simulink model "ERES_PIMC_Controller_Simulation"  (R2018a)
settings: Solver=VariableStepAuto  StartTime=0.0  StopTime=120  RelTol=1e-3
undefined symbols (not defined in the file): a_lateral_max, atableall, feedback_filter_limit_max, feedback_filter_limit_min, fl_x, fl_y, fr_x, fr_y, friction_table, imc_acc_error_coeffi, integrator_saturation_level, Ki, num, proportion, proportion_loop_limit, speed_controller_input_limit, station_error_limit, station_integrator_saturation_level, station_Ki, station_Kp, steer_angle_limited, steer_ratio, T7_with_trailer_atable, T7_with_trailer_atableall, T7_with_trailer_engine_speed_table, T7_with_trailer_engine_throttle_table, T7_with_trailer_engine_torqe_tableall, T7_with_trailer_utable, T7_with_trailer_utableall, T7_with_trailer_vtable, t_delay, throttle_table, utable, v_table, Vr, vtable, w1, w2, wheel_base, x0, y0
libraries: simulink x2, Solver_SF x1
(part 1 of 2)
settings Model: SimulationMode=rapid-accelerator  Creator=DELL  LastModifiedBy=DELL

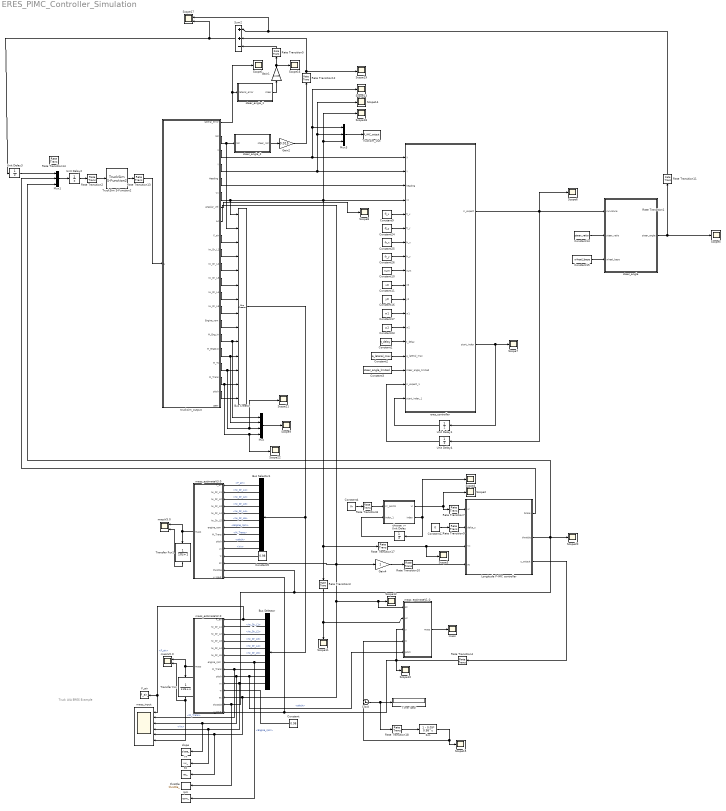
== system ERES_PIMC_Controller_Simulation ==
  note: Truck LKA ERES Example
  Bus Creator : BusCreator  Inputs=14
  Bus Selector : BusSelector  OutputSignals=F_air,Iw_Dr_L1,Iw_Dr_L2,Iw_Dr_L3,Iw_Dr_L4,Iw_Dr_L5,Engine_rpm,M_Trans,pitch,Vx
  Bus Selector1 : BusSelector  OutputSignals=F_air,Iw_Dr_L1,Iw_Dr_L2,Iw_Dr_L3,Iw_Dr_L4,Iw_Dr_L5,Engine_rpm,M_Trans,pitch,Vx
  Clock : Clock
  Constant : Constant  Value=0.98
  Constant1 : Constant  Value=t_delay
  Constant10 : Constant  Value=num
  Constant11 : Constant  Value=x0
  Constant12 : Constant  Value=0
  Constant14 : Constant  Value=steer_ratio
  Constant15 : Constant  Value=wheel_base
  Constant16 : Constant  Value=y0
  Constant17 : Constant  Value=w1
  Constant2 : Constant  Value=a_lateral_max
  Constant23 : Constant  Value=w2
  Constant24 : Constant  Value=fl_y
  Constant25 : Constant  Value=fr_x
  Constant26 : Constant  Value=fr_y
  Constant3 : Constant  Value=steer_angle_limited
  Constant4 : Constant  Value=Vr
  Constant5 : Constant  Value=0.98
  Constant9 : Constant  Value=fl_x
  F_air : ToWorkspace  VariableName=F_air_  SampleTime=0.01
  Fcn : Fcn  Expr=1 - 0.05* 0.98^u
  Gain1 : Gain  Gain=0.009
  Gain2 : Gain  Gain=0.015
  Gain4 : Gain
  Longitude P-IMC controller : Subsystem
  Mux : Mux
  Mux1 : Mux  Inputs=3
  Mux3 : Mux  Inputs=3
  Rate Transition{1,3..5,7..14,17..18} (14 alike) : RateTransition  OutPortSampleTime=0.01
  Rate Transition2 : RateTransition  OutPortSampleTime=0.001
  Scope{1..16,18..22} (21 alike) : Scope
  Scope17 : Scope  NumInputPorts=2
  Sum2 : Sum  Inputs=++-
  Time (sec) : Display
      settings: Format=bank  Decimation=100
  Transfer Fcn : TransferFcn  Denominator=[10 1]
  Transfer Fcn1 : TransferFcn  Denominator=[10 1]
  TruckSim S-Function2 : Solver_SF/TruckSim S-Function2  Priority=1  VehicleCode=s_ss__sss  SIMFILE=simfile.sim
      settings: AttributesFormatString=Vehicle Code: %<VehicleCode>
  Trucksim_Out : ToWorkspace  VariableName=P_IMC_output  SampleTime=-1
  Unit Delay : UnitDelay  InitialCondition=1  SampleTime=-1
  Unit Delay{1..4} (4 alike) : UnitDelay  SampleTime=0.01
  ac : ToWorkspace  VariableName=ac_  SampleTime=0.01
  choose_vr : MATLAB Function  TreatAsAtomicUnit=on
  eres_controller : MATLAB Function  TreatAsAtomicUnit=on
  mass : Scope
  massV2.0 : Scope  NumInputPorts=2
  massV3.0 : Scope  NumInputPorts=2
  mass_estimateV1.0 : Subsystem
  mass_estimateV2.0 : Subsystem
  mass_estimateV3.0 : Subsystem
  mass_input : Scope  NumInputPorts=6
  rpm : ToWorkspace  VariableName=rpm_  SampleTime=0.01
  slope : ToWorkspace  VariableName=slope_  SampleTime=0.01
  steer_angle : MATLAB Function  TreatAsAtomicUnit=on
  steer_angle_1 : Subsystem
  steer_angle_2 : Subsystem
  throttle : ToWorkspace  VariableName=throttle_  SampleTime=0.01
  trucksim_output : MATLAB Function  TreatAsAtomicUnit=on
  vx : ToWorkspace  VariableName=vx_  SampleTime=0.01
  wires:
  Constant1/1 -> eres_controller/14(t_delay)
  Constant3/1 -> eres_controller/16(steer_angle_limited)
  Unit Delay4/1 -> eres_controller/17(K_expect_1)
  TruckSim S-Function2/1 -> Rate Transition13/1
  Constant9/1 -> eres_controller/5(fl_x)
  Constant11/1 -> eres_controller/10(x0)
  eres_controller/2(start_index) -> Unit Delay1/1, Scope7/1
  Mux1/1 -> Unit Delay2/1
  Constant24/1 -> eres_controller/6(fl_y)
  Constant23/1 -> eres_controller/13(w2)
  Clock/1 -> Rate Transition18/1, Time (sec)/1
  Rate Transition8/1 -> choose_vr/1(Vr_points)
  Rate Transition7/1 -> Longitude P-IMC controller/1(vr)
  Unit Delay1/1 -> eres_controller/18(start_index_1)
  choose_vr/1(vr) -> Scope2/1, Rate Transition7/1
  Constant15/1 -> steer_angle/3(wheel_base)
  trucksim_output/8(Ac) -> mass_estimateV3.0/12(ac), mass_estimateV1.0/1(ac), Scope12/1, ac/1, mass_input/5, mass_estimateV2.0/12(ac), Gain4/1
  choose_vr/2(index) -> Unit Delay/1, Scope4/1
  Constant16/1 -> eres_controller/11(y0)
  Longitude P-IMC controller/2(throttle) -> throttle/1, mass_estimateV2.0/13(throttle), mass_estimateV3.0/13(throttle), Mux1/3, Scope20/1
  Constant25/1 -> eres_controller/7(fr_x)
  Constant4/1 -> Rate Transition8/1
  Rate Transition3/1 -> Scope11/1, mass_estimateV1.0/2(vc)
  Constant10/1 -> eres_controller/9(num)
  Longitude P-IMC controller/1(brake) -> Mux1/2
  Rate Transition18/1 -> Fcn/1
  Longitude P-IMC controller/3(u_output) -> Rate Transition4/1
  Rate Transition9/1 -> Longitude P-IMC controller/2(delta_s)
  Rate Transition13/1 -> trucksim_output/1(u)
  Constant17/1 -> eres_controller/12(w1)
  Unit Delay2/1 -> Rate Transition2/1
  Constant26/1 -> eres_controller/8(fr_y)
  Rate Transition2/1 -> TruckSim S-Function2/1
  eres_controller/1(K_expect) -> Scope6/1, steer_angle/1(curvature), Unit Delay4/1
  Constant14/1 -> steer_angle/2(steer_ratio)
  Rate Transition4/1 -> mass_estimateV3.0/14(u_input), mass_estimateV2.0/14(u_input), mass_estimateV1.0/3(u), Scope10/1
  trucksim_output/6(Vx) -> Bus Creator/1, Rate Transition17/1, Rate Transition3/1, Scope18/1, Mux3/3, eres_controller/4(vx)
  mass_estimateV1.0/1(mass) -> mass/1
  Rate Transition17/1 -> Longitude P-IMC controller/3(Vx), Scope3/1
  Constant12/1 -> Rate Transition9/1
  Unit Delay/1 -> choose_vr/2(index_1)
  Constant2/1 -> eres_controller/15(a_lateral_max)
  trucksim_output/7(angular_vel) -> Scope8/1
  Gain4/1 -> Rate Transition10/1
  steer_angle/1(steer_angle) -> Scope5/1, Rate Transition11/1
  Unit Delay3/1 -> Mux1/1
  Rate Transition10/1 -> Longitude P-IMC controller/4(ac)
  Mux3/1 -> Trucksim_Out/1
  trucksim_output/5(Heading) -> eres_controller/3(heading)
  trucksim_output/3(X) -> Mux3/1, Scope13/1, eres_controller/1(X)
  trucksim_output/4(Y) -> Mux3/2, Scope14/1, eres_controller/2(Y)
  trucksim_output/1(lateral_error) -> Scope1/1, steer_angle_1/1(lateral_error)
  Rate Transition5/1 -> Sum2/3
  Rate Transition11/1 -> Scope17/1, Sum2/1
  Sum2/1 -> Unit Delay3/1, Scope17/2
  steer_angle_1/1(steer) -> Gain1/1
  Gain1/1 -> Scope16/1, Rate Transition5/1
  trucksim_output/2(roll) -> Bus Creator/2, steer_angle_2/1(roll)
  steer_angle_2/1(steer_roll) -> Gain2/1
  Rate Transition12/1 -> Scope19/1, Sum2/2
  Gain2/1 -> Rate Transition12/1
  trucksim_output/19(M_Trans) -> Scope22/1, Mux/4, Bus Creator/13
  trucksim_output/18(M_Tc) -> Scope21/1, Mux/3, Bus Creator/12
  trucksim_output/17(M_EngOut) -> Mux/2, Bus Creator/11
  trucksim_output/16(M_Eng_In) -> Mux/1, Bus Creator/10
  trucksim_output/15(Engine_rpm) -> Bus Creator/9
  trucksim_output/14(Iw_Dr_L5) -> Bus Creator/8
  trucksim_output/13(Iw_Dr_L4) -> Bus Creator/7
  trucksim_output/12(Iw_Dr_L3) -> Bus Creator/6
  trucksim_output/11(Iw_Dr_L2) -> Bus Creator/5
  trucksim_output/10(Iw_Dr_L1) -> Bus Creator/4
  trucksim_output/9(F_air) -> Bus Creator/3
  Bus Creator/1 -> Bus Selector/1, Bus Selector1/1
  Bus Selector/1 -> F_air/1, mass_input/1, mass_estimateV2.0/1(F_air)  "<F_air>"
  Bus Selector/2 -> mass_estimateV2.0/2(Iw_Dr_L1)  "<Iw_Dr_L1>"
  Bus Selector/3 -> mass_estimateV2.0/3(Iw_Dr_L2)  "<Iw_Dr_L2>"
  Bus Selector/4 -> mass_estimateV2.0/4(Iw_Dr_L3)  "<Iw_Dr_L3>"
  Bus Selector/5 -> mass_estimateV2.0/5(Iw_Dr_L4)  "<Iw_Dr_L4>"
  Bus Selector/6 -> mass_estimateV2.0/6(Iw_Dr_L5)  "<Iw_Dr_L5>"
  Bus Selector/7 -> rpm/1, mass_estimateV2.0/7(engine_rpm)  "<Engine_rpm>"
  Bus Selector/8 -> mass_input/2, mass_estimateV2.0/8(M_Trans)  "<M_Trans>"
  Bus Selector/9 -> mass_estimateV1.0/5(pitch), slope/1, mass_input/3, mass_estimateV2.0/9(pitch)  "<pitch>"
  Bus Selector/10 -> vx/1, mass_input/4, mass_estimateV2.0/10(vx)  "<Vx>"
  Fcn/1 -> Scope15/1, mass_estimateV1.0/4(w)
  mass_estimateV2.0/1(mass) -> massV2.0/1, Transfer Fcn/1
  trucksim_output/20(pitch) -> Bus Creator/14
  Mux/1 -> Scope9/1
  Transfer Fcn/1 -> massV2.0/2, mass_input/6
  Constant/1 -> mass_estimateV2.0/11(w)
  Bus Selector1/1 -> mass_estimateV3.0/1(F_air)  "<F_air>"
  Bus Selector1/2 -> mass_estimateV3.0/2(Iw_Dr_L1)  "<Iw_Dr_L1>"
  Bus Selector1/3 -> mass_estimateV3.0/3(Iw_Dr_L2)  "<Iw_Dr_L2>"
  Bus Selector1/4 -> mass_estimateV3.0/4(Iw_Dr_L3)  "<Iw_Dr_L3>"
  Bus Selector1/5 -> mass_estimateV3.0/5(Iw_Dr_L4)  "<Iw_Dr_L4>"
  Bus Selector1/6 -> mass_estimateV3.0/6(Iw_Dr_L5)  "<Iw_Dr_L5>"
  Bus Selector1/7 -> mass_estimateV3.0/7(engine_rpm)  "<Engine_rpm>"
  Bus Selector1/8 -> mass_estimateV3.0/8(M_Trans)  "<M_Trans>"
  Bus Selector1/9 -> mass_estimateV3.0/9(pitch)  "<pitch>"
  Bus Selector1/10 -> mass_estimateV3.0/10(vx)  "<Vx>"
  Constant5/1 -> mass_estimateV3.0/11(w)
  Transfer Fcn1/1 -> massV3.0/2
  mass_estimateV3.0/1(mass) -> Transfer Fcn1/1, massV3.0/1

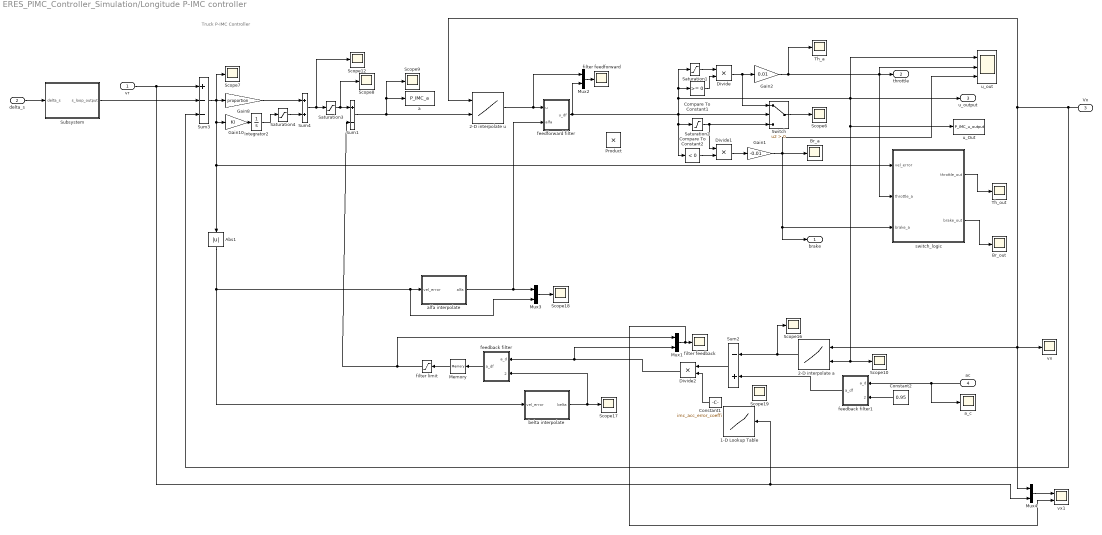
== system ERES_PIMC_Controller_Simulation/Longitude P-IMC controller ==
  note: Truck P-IMC Controller
  vr : Inport
  delta_s : Inport  Port=2
  Vx : Inport  Port=3
  ac : Inport  Port=4
  1-D Lookup Table : Lookup_n-D  NumberOfTableDimensions=1  BreakpointsForDimension1=[5 8 15 20 25 30]  Table=[0.3 0.45 0.65 0.8 0.9 1.0]  InternalRulePriority=Speed  RndMeth=Simplest  InputSameDT=on
  2-D interpolate a : Lookup_n-D  BreakpointsForDimension1=T7_with_trailer_vtable  BreakpointsForDimension2=T7_with_trailer_utable  Table=T7_with_trailer_atableall  ExtrapMethod=Clip  InternalRulePriority=Speed  RndMeth=Simplest  InputSameDT=on
  2-D interpolate u : Lookup_n-D  BreakpointsForDimension1=T7_with_trailer_vtable  BreakpointsForDimension2=T7_with_trailer_atable  Table=T7_with_trailer_utableall  ExtrapMethod=Clip  InternalRulePriority=Speed  RndMeth=Simplest  InputSameDT=on
  Abs1 : Abs
  Br_a : Scope
  Br_out : Scope
  Compare To Constant1 : simulink/Logic and Bit Operations/Compare To Constant  relop=>=  const=0  OutDataTypeStr=boolean
  Compare To Constant2 : simulink/Logic and Bit Operations/Compare To Constant  relop=<  const=0  OutDataTypeStr=boolean
  Constant1 : Constant  Value=imc_acc_error_coeffi
  Constant2 : Constant  Value=0.95
  Divide : Product  Inputs=**
  Divide1 : Product  Inputs=**
  Divide2 : Product  Inputs=**
  Gain1 : Gain  Gain=-0.01
  Gain10 : Gain  Gain=Ki
  Gain2 : Gain  Gain=0.01
  Gain8 : Gain  Gain=proportion
  Integrator2 : Integrator
  Memory : Memory
  Mux{1..4} (4 alike) : Mux  Inputs=2
  Product : Product
  Saturation1 : Saturate  UpperLimit=90  LowerLimit=0
  Saturation2 : Saturate  UpperLimit=0  LowerLimit=-60
  Saturation3 : Saturate  UpperLimit=proportion_loop_limit  LowerLimit=-proportion_loop_limit
  Saturation4 : Saturate  UpperLimit=integrator_saturation_level  LowerLimit=-integrator_saturation_level
  Scope{6..10,12,16..19} (10 alike) : Scope
  Subsystem : Subsystem
  Sum1 : Sum  Inputs=+-
  Sum2 : Sum  Inputs=-+
  Sum3 : Sum  Inputs=+--
  Sum4 : Sum
  Switch : Switch  Criteria=u2 > Threshold
  Th_a : Scope
  Th_out : Scope
  a : ToWorkspace  VariableName=P_IMC_a  SampleTime=0.01
  a_c : Scope
  alfa interpolate : MATLAB Function  TreatAsAtomicUnit=on
  belta interpolate : MATLAB Function  TreatAsAtomicUnit=on
  feedback filter : Subsystem
  feedback filter1 : Subsystem
  feedforward filter : Subsystem
  filter feedback : Scope
  filter feedforward : Scope
  filter limit : Saturate  UpperLimit=feedback_filter_limit_max  LowerLimit=feedback_filter_limit_min
  switch_logic : Subsystem
  u_Out : ToWorkspace  VariableName=P_IMC_u_output  SampleTime=0.01
  u_out : Scope  NumInputPorts=3
  vx : Scope
  vx1 : Scope  NumInputPorts=2
  brake : Outport
  throttle : Outport  Port=2
  u_output : Outport  Port=3
  wires:
  Vx/1 -> 2-D interpolate u/1, Mux4/1, 2-D interpolate a/1, vx/1, Sum3/3
  Sum1/1 -> a/1, Scope9/1, 2-D interpolate u/2
  Divide1/1 -> Gain1/1
  Compare To Constant2/1 -> Divide1/2
  Divide/1 -> Switch/1, Gain2/1
  Compare To Constant1/1 -> Divide/2
  Saturation1/1 -> Divide/1
  2-D interpolate u/1 -> Mux2/1, feedforward filter/1(u)
  Gain1/1 -> u_out/3, switch_logic/3(brake_a), brake/1, Br_a/1
  Gain2/1 -> u_out/2, throttle/1, switch_logic/2(throttle_a), Th_a/1
  Switch/1 -> Scope6/1
  Saturation2/1 -> Switch/3, Divide1/1
  Sum3/1 -> Gain8/1, Scope7/1, Gain10/1, switch_logic/1(vel_error), Abs1/1
  Saturation3/1 -> Scope8/1, Sum1/1
  delta_s/1 -> Subsystem/1(delta_s)
  Subsystem/1(s_loop_output) -> Sum3/2
  ac/1 -> a_c/1, feedback filter1/1(a_d)
  Sum4/1 -> Scope12/1, Saturation3/1
  Gain8/1 -> Sum4/1
  Gain10/1 -> Integrator2/1
  Mux1/1 -> vx1/2, filter feedback/1
  feedback filter/1(a_df) -> Memory/1
  Memory/1 -> filter limit/1
  2-D interpolate a/1 -> Sum2/1, Scope16/1
  filter limit/1 -> Sum1/2, Mux1/1
  alfa interpolate/1(alfa) -> Mux3/1, feedforward filter/2(alfa)
  Abs1/1 -> Mux3/2, alfa interpolate/1(vel_error), belta interpolate/1(vel_error)
  Mux3/1 -> Scope18/1
  Mux2/1 -> filter feedforward/1
  belta interpolate/1(belta) -> feedback filter/2(belta), Scope17/1
  vr/1 -> 1-D Lookup Table/1, Mux4/2, Sum3/1
  Sum2/1 -> Divide2/1
  Divide2/1 -> Mux1/2, feedback filter/1(a_d)
  feedforward filter/1(u_df) -> Compare To Constant1/1, Saturation1/1, u_out/1, u_Out/1, Scope10/1, 2-D interpolate a/2, u_output/1, Saturation2/1, Compare To Constant2/1, Switch/2, Mux2/2
  switch_logic/1(throttle_out) -> Th_out/1
  switch_logic/2(brake_out) -> Br_out/1
  Constant2/1 -> feedback filter1/2(belta)
  feedback filter1/1(a_df) -> Sum2/2
  Mux4/1 -> vx1/1
  Integrator2/1 -> Saturation4/1
  Saturation4/1 -> Sum4/2
  Constant1/1 -> Divide2/2

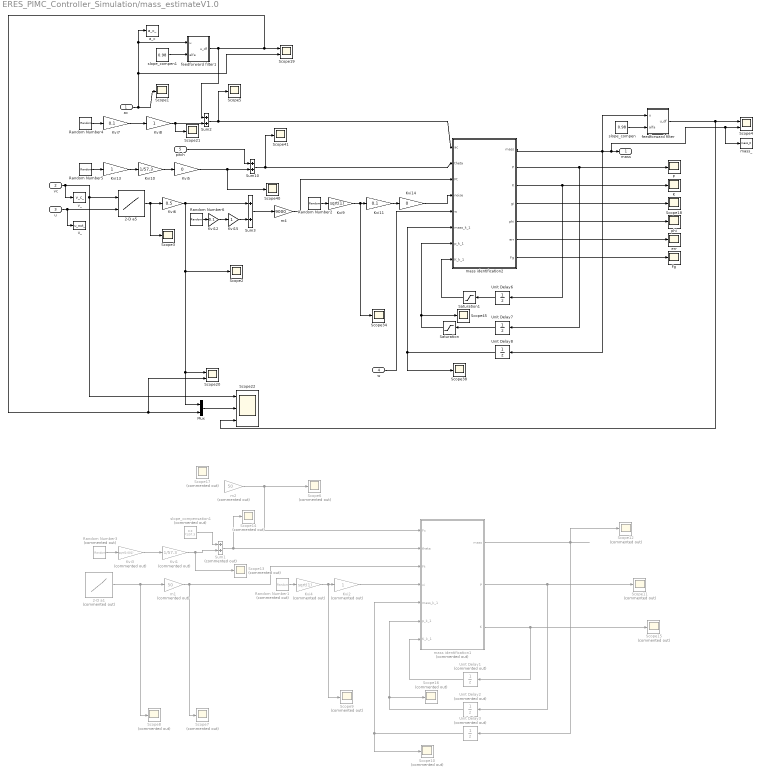
== system ERES_PIMC_Controller_Simulation/mass_estimateV1.0 ==
  ac : Inport
  vc : Inport  Port=2
  u : Inport  Port=3
  w : Inport  Port=4
  pitch : Inport  Port=5
  2-D a1 : Lookup_n-D  Commented=on  BreakpointsForDimension1=vtable  BreakpointsForDimension2=utable  BreakpointsForDimension3=[-60 -50]  Table=atableall  InternalRulePriority=Speed  RndMeth=Simplest  InputSameDT=on
  2-D a5 : Lookup_n-D  BreakpointsForDimension1=T7_with_trailer_vtable  BreakpointsForDimension2=T7_with_trailer_utable  BreakpointsForDimension3=[-60 -50]  Table=T7_with_trailer_atableall  InternalRulePriority=Speed  RndMeth=Simplest  InputSameDT=on
  Fg : Scope
  K : Scope
  Kvi1 : Gain  Commented=on  Gain=1/57.3
  Kvi10 : Gain  Gain=1/57.3
  Kvi11 : Gain  Gain=0.1
  Kvi12 : Gain  Gain=0.1
  Kvi13 : Gain
  Kvi14 : Gain  Gain=0
  Kvi15 : Gain
  Kvi2 : Gain  Commented=on
  Kvi3 : Gain  Commented=on  Gain=sqrt(0.001)
  Kvi4 : Gain  Commented=on  Gain=sqrt(1)
  Kvi5 : Gain  Gain=0
  Kvi6 : Gain  Gain=0.5
  Kvi7 : Gain  Gain=0.1
  Kvi8 : Gain
  Kvi9 : Gain  Gain=sqrt(1)
  Mux : Mux  Inputs=2
  P : Scope
  Random Number1 : RandomNumber  Commented=on  SampleTime=0.01
  Random Number{2,4..6} (4 alike) : RandomNumber  SampleTime=0.01
  Random Number3 : RandomNumber  Commented=on  Variance=0.1  SampleTime=0.01
  Saturation : Saturate  UpperLimit=10000000  LowerLimit=0.02
  Saturation1 : Saturate  UpperLimit=100  LowerLimit=0.1
  Scope{1..3,5,18,21,34,38,40..41,45} (11 alike) : Scope
  Scope{6..17} (12 alike) : Scope  Commented=on
  Scope19 : Scope  NumInputPorts=2
  Scope20 : Scope  NumInputPorts=2
  Scope22 : Scope  NumInputPorts=3
  Scope4 : Scope  NumInputPorts=2
  Sum1 : Sum  Commented=on
  Sum10 : Sum
  Sum2 : Sum
  Sum3 : Sum
  Unit Delay1 : UnitDelay  Commented=on  InitialCondition=1  SampleTime=0.01
  Unit Delay2 : UnitDelay  Commented=on  InitialCondition=100000  SampleTime=0.01
  Unit Delay3 : UnitDelay  Commented=on  InitialCondition=30000  SampleTime=0.01
  Unit Delay6 : UnitDelay  InitialCondition=10  SampleTime=0.01
  Unit Delay7 : UnitDelay  InitialCondition=100000  SampleTime=0.01
  Unit Delay8 : UnitDelay  InitialCondition=40000  SampleTime=0.01
  a_c : ToWorkspace  VariableName=a_c_  SampleTime=0.01
  err : Scope
  feedforward filter : Subsystem
  feedforward filter1 : Subsystem
  m1 : Gain  Commented=on  Gain=50
  m2 : Gain  Commented=on  Gain=50
  m4 : Gain  Gain=9000
  mass identification1 : MATLAB Function  Commented=on  TreatAsAtomicUnit=on  SystemSampleTime=0.01
  mass identification2 : MATLAB Function  TreatAsAtomicUnit=on  SystemSampleTime=0.01
  mass_ : ToWorkspace  VariableName=mass_0  SampleTime=0.01
  phi : Scope
  slope_compen : Constant  Value=0.98
  slope_compen1 : Constant  Value=0.98
  slope_compensation1 : Constant  Commented=on  Value=0.0 *1/57.3
  u_ : ToWorkspace  VariableName=u_out_  SampleTime=0.01
  v_ : ToWorkspace  VariableName=v_c_  SampleTime=0.01
  mass : Outport
  wires:
  Unit Delay7/1 -> Saturation/1
  mass identification2/1(mass) -> feedforward filter/1(u), Unit Delay8/1, mass_/1, Scope4/2, mass/1
  mass identification2/3(K) -> Unit Delay6/1, K/1
  Unit Delay6/1 -> Saturation1/1
  Kvi13/1 -> Kvi10/1
  Kvi11/1 -> Kvi14/1
  Random Number2/1 -> Kvi9/1
  Unit Delay8/1 -> mass identification2/6(mass_k_1), Scope38/1
  pitch/1 -> Sum10/1
  Kvi10/1 -> Kvi5/1
  Random Number5/1 -> Kvi13/1
  mass identification2/2(P) -> Unit Delay7/1, P/1
  vc/1 -> v_/1, Scope22/1, 2-D a5/1
  Kvi9/1 -> Kvi11/1, Scope34/1
  Sum10/1 -> mass identification2/2(theta), Scope41/1
  u/1 -> u_/1, 2-D a5/2
  m2/1 -> Scope6/1, mass identification1/1(Fc)
  ? -> 2-D a1/2
  m1/1 -> mass identification1/3(Ft), Scope7/1
  Sum1/1 -> Scope14/1, mass identification1/2(theta)
  Kvi4/1 -> Scope9/1, Kvi2/1
  ? -> 2-D a1/1
  2-D a1/1 -> m1/1, Scope8/1
  mass identification1/2(P) -> Scope11/1, Unit Delay2/1
  Random Number3/1 -> Kvi3/1
  Kvi1/1 -> Scope13/1, Sum1/2
  slope_compensation1/1 -> Sum1/1
  Unit Delay3/1 -> Scope10/1, mass identification1/5(mass_k_1)
  Random Number1/1 -> Kvi4/1
  Kvi2/1 -> mass identification1/4(xi)
  ? -> m2/1, Scope17/1
  Kvi3/1 -> Kvi1/1
  Unit Delay1/1 -> mass identification1/7(K_k_1)
  mass identification1/3(K) -> Scope15/1, Unit Delay1/1
  mass identification1/1(mass) -> Unit Delay3/1, Scope12/1
  Unit Delay2/1 -> Scope16/1, mass identification1/6(p_k_1)
  mass identification2/4(gi) -> Scope18/1
  mass identification2/5(phi) -> phi/1
  Kvi5/1 -> Scope40/1, Sum10/2
  Random Number4/1 -> Kvi7/1
  Kvi7/1 -> Kvi8/1
  Kvi8/1 -> Scope21/1, Sum2/2
  w/1 -> mass identification2/5(w)
  feedforward filter/1(u_df) -> Scope22/3, Scope4/1
  slope_compen/1 -> feedforward filter/2(alfa)
  2-D a5/1 -> Scope3/1, Kvi6/1
  Sum2/1 -> mass identification2/1(ac), Scope5/1
  mass identification2/6(err) -> err/1
  Saturation/1 -> mass identification2/7(p_k_1), Scope45/1
  Saturation1/1 -> mass identification2/8(K_k_1)
  slope_compen1/1 -> feedforward filter1/2(alfa)
  feedforward filter1/1(u_df) -> Sum2/1, Scope20/2, Mux/2, Scope19/1
  ac/1 -> Scope1/1, Scope19/2, feedforward filter1/1(u), a_c/1
  Mux/1 -> Scope22/2
  Random Number6/1 -> Kvi12/1
  Kvi12/1 -> Kvi15/1
  Sum3/1 -> m4/1
  Kvi6/1 -> Scope2/1, Scope20/1, Mux/1, Sum3/1
  m4/1 -> mass identification2/3(Ft)
  mass identification2/7(Fg) -> Fg/1
  Kvi14/1 -> mass identification2/4(noise)
  Kvi15/1 -> Sum3/2

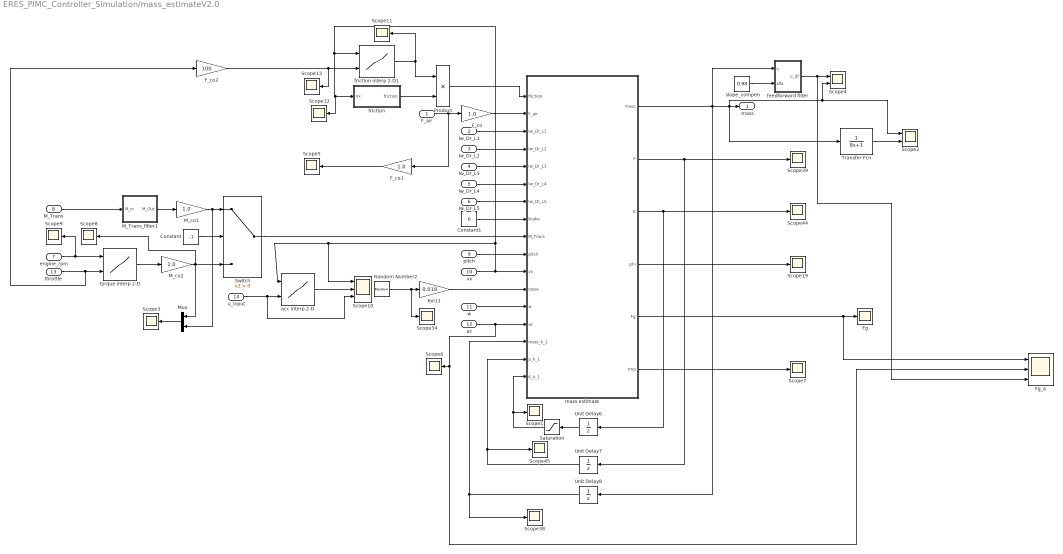
== system ERES_PIMC_Controller_Simulation/mass_estimateV2.0 ==
  F_air : Inport
  Iw_Dr_L1 : Inport  Port=2
  Iw_Dr_L2 : Inport  Port=3
  Iw_Dr_L3 : Inport  Port=4
  Iw_Dr_L4 : Inport  Port=5
  Iw_Dr_L5 : Inport  Port=6
  engine_rpm : Inport  Port=7
  M_Trans : Inport  Port=8
  pitch : Inport  Port=9
  vx : Inport  Port=10
  w : Inport  Port=11
  ac : Inport  Port=12
  throttle : Inport  Port=13
  u_input : Inport  Port=14
  Constant : Constant  Value=-1
  Constant1 : Constant  Value=0
  F_co : Gain  Gain=1.0
  F_co1 : Gain  Gain=1.0
  F_co2 : Gain  Gain=100
  Fg : Scope
  Fg_a : Scope  NumInputPorts=3
  Kvi11 : Gain  Gain=0.018
  M_Trans_filter1 : Subsystem
  M_co1 : Gain  Gain=1.0
  M_co2 : Gain  Gain=1.0
  Mux : Mux  Inputs=2
  Product : Product
  Random Number2 : RandomNumber  SampleTime=0.01
  Saturation : Saturate  UpperLimit=10  LowerLimit=0.01
  Scope{1,3,5..9,11..13,19,34,38..39,44..45} (16 alike) : Scope
  Scope10 : Scope  NumInputPorts=3
  Scope2 : Scope  NumInputPorts=2
  Scope4 : Scope  NumInputPorts=2
  Switch : Switch  Criteria=u2 > Threshold
  Transfer Fcn : TransferFcn  Denominator=[8 1]
  Unit Delay6 : UnitDelay  SampleTime=0.01
  Unit Delay7 : UnitDelay  InitialCondition=1000000  SampleTime=0.01
  Unit Delay8 : UnitDelay  InitialCondition=40000  SampleTime=0.01
  acc interp 2-D : Lookup_n-D  BreakpointsForDimension1=T7_with_trailer_vtable  BreakpointsForDimension2=T7_with_trailer_utable  BreakpointsForDimension3=[-60 -50]  Table=T7_with_trailer_atableall  InternalRulePriority=Speed  RndMeth=Simplest  InputSameDT=on
  feedforward filter : Subsystem
  friction : Subsystem
  friction interp 2-D1 : Lookup_n-D  BreakpointsForDimension1=v_table  BreakpointsForDimension2=throttle_table  BreakpointsForDimension3=[-60 -50]  Table=friction_table  InternalRulePriority=Speed  RndMeth=Simplest  InputSameDT=on
  mass estimate : MATLAB Function  TreatAsAtomicUnit=on  SystemSampleTime=0.01
  slope_compen : Constant  Value=0.98
  "torque interp 2-D " : Lookup_n-D  BreakpointsForDimension1=T7_with_trailer_engine_speed_table  BreakpointsForDimension2=T7_with_trailer_engine_throttle_table  BreakpointsForDimension3=[-60 -50]  Table=T7_with_trailer_engine_torqe_tableall  InternalRulePriority=Speed  RndMeth=Simplest  InputSameDT=on
  mass : Outport
  wires:
  slope_compen/1 -> feedforward filter/2(alfa)
  feedforward filter/1(u_df) -> Fg_a/3, Scope4/1
  mass estimate/4(phi) -> Scope19/1
  Random Number2/1 -> Scope34/1, Kvi11/1
  mass estimate/2(P) -> Unit Delay7/1, Scope39/1
  Unit Delay6/1 -> Saturation/1
  mass estimate/3(K) -> Unit Delay6/1, Scope44/1
  mass estimate/1(mass) -> Unit Delay8/1, Transfer Fcn/1, mass/1, Scope2/1, Scope4/2, feedforward filter/1(u)
  Unit Delay7/1 -> Scope45/1, mass estimate/16(p_k_1)
  Iw_Dr_L5/1 -> mass estimate/7(Iw_Dr_L5)
  Iw_Dr_L4/1 -> mass estimate/6(Iw_Dr_L4)
  Iw_Dr_L3/1 -> mass estimate/5(Iw_Dr_L3)
  Iw_Dr_L2/1 -> mass estimate/4(Iw_Dr_L2)
  Iw_Dr_L1/1 -> mass estimate/3(Iw_Dr_L1)
  F_air/1 -> F_co1/1, F_co/1
  w/1 -> mass estimate/13(w)
  vx/1 -> Scope10/1, acc interp 2-D/1, friction interp 2-D1/1, Scope12/1, friction/1(Vx), mass estimate/11(vx)
  ac/1 -> Fg_a/2, Scope6/1, mass estimate/14(ac)
  Unit Delay8/1 -> Scope38/1, mass estimate/15(mass_k_1)
  Saturation/1 -> Scope1/1, mass estimate/17(K_k_1)
  mass estimate/6(tmp) -> Scope7/1
  mass estimate/5(Fg) -> Fg_a/1, Fg/1
  pitch/1 -> mass estimate/10(pitch)
  Switch/1 -> mass estimate/9(M_Trans)
  F_co/1 -> mass estimate/2(F_air)
  friction/1(friction) -> Product/2
  Product/1 -> mass estimate/1(friction)
  Transfer Fcn/1 -> Scope2/2
  F_co1/1 -> Scope5/1
  Constant/1 -> Switch/2
  M_Trans_filter1/1(M_Out) -> M_co1/1
  M_co1/1 -> Mux/2, Switch/1
  "torque interp 2-D "/1 -> M_co2/1
  engine_rpm/1 -> Scope9/1, "torque interp 2-D "/1
  throttle/1 -> F_co2/1, "torque interp 2-D "/2
  M_Trans/1 -> M_Trans_filter1/1(M_in)
  M_co2/1 -> Scope8/1, Mux/1, Switch/3
  Mux/1 -> Scope3/1
  Constant1/1 -> mass estimate/8(brake)
  acc interp 2-D/1 -> Scope10/2
  u_input/1 -> Scope10/3, acc interp 2-D/2
  F_co2/1 -> friction interp 2-D1/2, Scope13/1
  friction interp 2-D1/1 -> Product/1, Scope11/1
  Kvi11/1 -> mass estimate/12(noise)

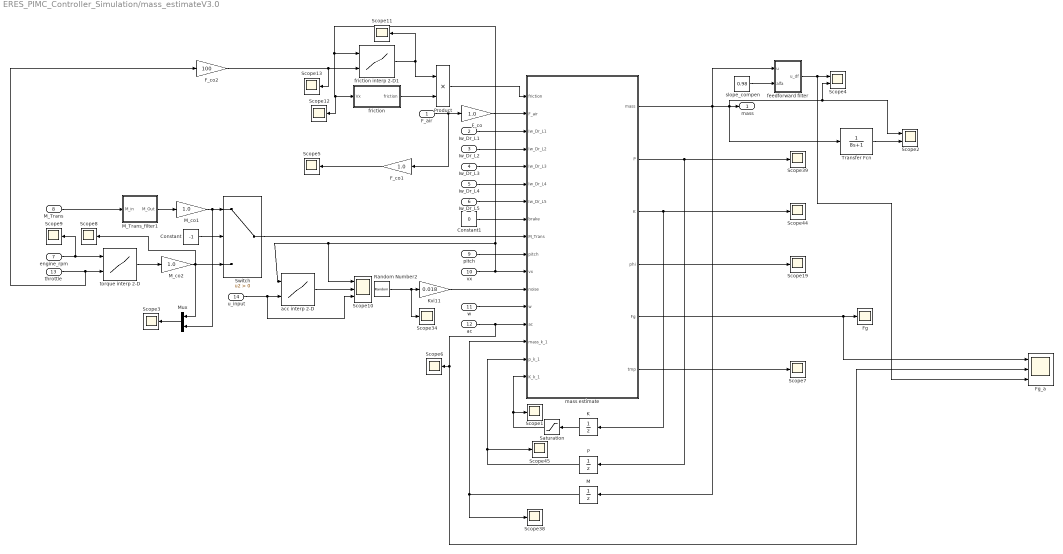
== system ERES_PIMC_Controller_Simulation/mass_estimateV3.0 ==
  F_air : Inport
  Iw_Dr_L1 : Inport  Port=2
  Iw_Dr_L2 : Inport  Port=3
  Iw_Dr_L3 : Inport  Port=4
  Iw_Dr_L4 : Inport  Port=5
  Iw_Dr_L5 : Inport  Port=6
  engine_rpm : Inport  Port=7
  M_Trans : Inport  Port=8
  pitch : Inport  Port=9
  vx : Inport  Port=10
  w : Inport  Port=11
  ac : Inport  Port=12
  throttle : Inport  Port=13
  u_input : Inport  Port=14
  Constant : Constant  Value=-1
  Constant1 : Constant  Value=0
  F_co : Gain  Gain=1.0
  F_co1 : Gain  Gain=1.0
  F_co2 : Gain  Gain=100
  Fg : Scope
  Fg_a : Scope  NumInputPorts=3
  K : UnitDelay  SampleTime=0.01
  Kvi11 : Gain  Gain=0.018
  M : UnitDelay  InitialCondition=40000  SampleTime=0.01
  M_Trans_filter1 : Subsystem
  M_co1 : Gain  Gain=1.0
  M_co2 : Gain  Gain=1.0
  Mux : Mux  Inputs=2
  P : UnitDelay  InitialCondition=1000000  SampleTime=0.01
  Product : Product
  Random Number2 : RandomNumber  SampleTime=0.01
  Saturation : Saturate  UpperLimit=10  LowerLimit=0.01
  Scope{1,3,5..9,11..13,19,34,38..39,44..45} (16 alike) : Scope
  Scope10 : Scope  NumInputPorts=3
  Scope2 : Scope  NumInputPorts=2
  Scope4 : Scope  NumInputPorts=2
  Switch : Switch  Criteria=u2 > Threshold
  Transfer Fcn : TransferFcn  Denominator=[8 1]
  acc interp 2-D : Lookup_n-D  BreakpointsForDimension1=T7_with_trailer_vtable  BreakpointsForDimension2=T7_with_trailer_utable  BreakpointsForDimension3=[-60 -50]  Table=T7_with_trailer_atableall  InternalRulePriority=Speed  RndMeth=Simplest  InputSameDT=on
  feedforward filter : Subsystem
  friction : Subsystem
  friction interp 2-D1 : Lookup_n-D  BreakpointsForDimension1=v_table  BreakpointsForDimension2=throttle_table  BreakpointsForDimension3=[-60 -50]  Table=friction_table  InternalRulePriority=Speed  RndMeth=Simplest  InputSameDT=on
  mass estimate : MATLAB Function  TreatAsAtomicUnit=on  SystemSampleTime=0.01
  slope_compen : Constant  Value=0.98
  "torque interp 2-D " : Lookup_n-D  BreakpointsForDimension1=T7_with_trailer_engine_speed_table  BreakpointsForDimension2=T7_with_trailer_engine_throttle_table  BreakpointsForDimension3=[-60 -50]  Table=T7_with_trailer_engine_torqe_tableall  InternalRulePriority=Speed  RndMeth=Simplest  InputSameDT=on
  mass : Outport
  wires:
  Kvi11/1 -> mass estimate/12(noise)
  friction interp 2-D1/1 -> Scope11/1, Product/1
  F_co2/1 -> Scope13/1, friction interp 2-D1/2
  u_input/1 -> acc interp 2-D/2, Scope10/3
  acc interp 2-D/1 -> Scope10/2
  Constant1/1 -> mass estimate/8(brake)
  Mux/1 -> Scope3/1
  M_co2/1 -> Switch/3, Mux/1, Scope8/1
  M_Trans/1 -> M_Trans_filter1/1(M_in)
  throttle/1 -> "torque interp 2-D "/2, F_co2/1
  engine_rpm/1 -> "torque interp 2-D "/1, Scope9/1
  "torque interp 2-D "/1 -> M_co2/1
  M_co1/1 -> Switch/1, Mux/2
  M_Trans_filter1/1(M_Out) -> M_co1/1
  Constant/1 -> Switch/2
  F_co1/1 -> Scope5/1
  Transfer Fcn/1 -> Scope2/2
  Product/1 -> mass estimate/1(friction)
  friction/1(friction) -> Product/2
  F_co/1 -> mass estimate/2(F_air)
  Switch/1 -> mass estimate/9(M_Trans)
  pitch/1 -> mass estimate/10(pitch)
  mass estimate/5(Fg) -> Fg/1, Fg_a/1
  mass estimate/6(tmp) -> Scope7/1
  Saturation/1 -> mass estimate/17(K_k_1), Scope1/1
  M/1 -> mass estimate/15(mass_k_1), Scope38/1
  ac/1 -> mass estimate/14(ac), Scope6/1, Fg_a/2
  vx/1 -> mass estimate/11(vx), friction/1(Vx), Scope12/1, friction interp 2-D1/1, acc interp 2-D/1, Scope10/1
  w/1 -> mass estimate/13(w)
  F_air/1 -> F_co/1, F_co1/1
  Iw_Dr_L1/1 -> mass estimate/3(Iw_Dr_L1)
  Iw_Dr_L2/1 -> mass estimate/4(Iw_Dr_L2)
  Iw_Dr_L3/1 -> mass estimate/5(Iw_Dr_L3)
  Iw_Dr_L4/1 -> mass estimate/6(Iw_Dr_L4)
  Iw_Dr_L5/1 -> mass estimate/7(Iw_Dr_L5)
  P/1 -> mass estimate/16(p_k_1), Scope45/1
  mass estimate/1(mass) -> feedforward filter/1(u), Scope4/2, Scope2/1, mass/1, Transfer Fcn/1, M/1
  mass estimate/3(K) -> Scope44/1, K/1
  K/1 -> Saturation/1
  mass estimate/2(P) -> Scope39/1, P/1
  Random Number2/1 -> Kvi11/1, Scope34/1
  mass estimate/4(phi) -> Scope19/1
  feedforward filter/1(u_df) -> Scope4/1, Fg_a/3
  slope_compen/1 -> feedforward filter/2(alfa)

== system ERES_PIMC_Controller_Simulation/steer_angle_1 ==
  lateral_error : Inport
  steer_compensation : MATLAB Function  TreatAsAtomicUnit=on
  steer : Outport
  wires:
  lateral_error/1 -> steer_compensation/1(lateral_error)
  steer_compensation/1(steer_compensation) -> steer/1

== system ERES_PIMC_Controller_Simulation/steer_angle_2 ==
  roll : Inport
  steer_roll_compensation : MATLAB Function  TreatAsAtomicUnit=on
  steer_roll : Outport
  wires:
  steer_roll_compensation/1(steer_roll_) -> steer_roll/1
  roll/1 -> steer_roll_compensation/1(roll)

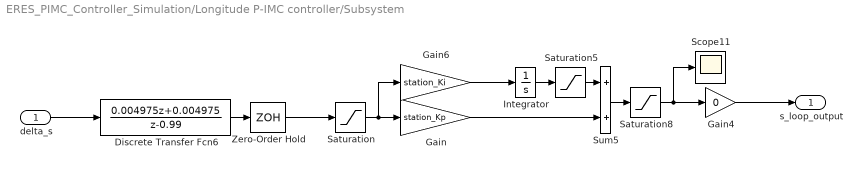
== system ERES_PIMC_Controller_Simulation/Longitude P-IMC controller/Subsystem ==
  delta_s : Inport
  Discrete Transfer Fcn6 : DiscreteTransferFcn  Numerator=[0.004975 0.004975]  Denominator=[1 -0.99]
  Gain : Gain  Gain=station_Kp
  Gain4 : Gain  Gain=0
  Gain6 : Gain  Gain=station_Ki
  Integrator : Integrator
  Saturation : Saturate  UpperLimit=station_error_limit  LowerLimit=-station_error_limit
  Saturation5 : Saturate  UpperLimit=station_integrator_saturation_level  LowerLimit=-station_integrator_saturation_level
  Saturation8 : Saturate  UpperLimit=speed_controller_input_limit  LowerLimit=-speed_controller_input_limit
  Scope11 : Scope
  Sum5 : Sum
  Zero-Order Hold : ZeroOrderHold  SampleTime=0.01
  s_loop_output : Outport
  wires:
  Sum5/1 -> Saturation8/1
  Gain6/1 -> Integrator/1
  Gain/1 -> Sum5/2
  Discrete Transfer Fcn6/1 -> Zero-Order Hold/1
  Saturation5/1 -> Sum5/1
  Saturation8/1 -> Gain4/1, Scope11/1
  Saturation/1 -> Gain/1, Gain6/1
  delta_s/1 -> Discrete Transfer Fcn6/1
  Integrator/1 -> Saturation5/1
  Zero-Order Hold/1 -> Saturation/1
  Gain4/1 -> s_loop_output/1

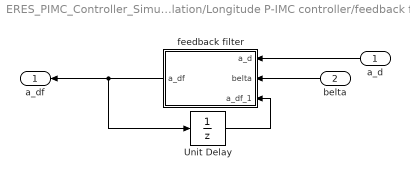
== system ERES_PIMC_Controller_Simulation/Longitude P-IMC controller/feedback filter ==
  a_d : Inport
  belta : Inport  Port=2
  Unit Delay : UnitDelay  SampleTime=-1
  feedback filter : MATLAB Function  TreatAsAtomicUnit=on
  a_df : Outport
  wires:
  Unit Delay/1 -> feedback filter/3(a_df_1)
  a_d/1 -> feedback filter/1(a_d)
  feedback filter/1(a_df) -> a_df/1, Unit Delay/1
  belta/1 -> feedback filter/2(belta)

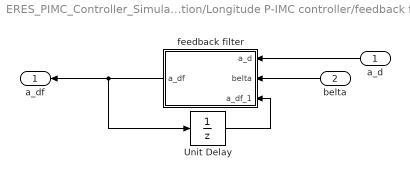
== system ERES_PIMC_Controller_Simulation/Longitude P-IMC controller/feedback filter1 ==
  a_d : Inport
  belta : Inport  Port=2
  Unit Delay : UnitDelay  SampleTime=-1
  feedback filter : MATLAB Function  TreatAsAtomicUnit=on
  a_df : Outport
  wires:
  belta/1 -> feedback filter/2(belta)
  feedback filter/1(a_df) -> Unit Delay/1, a_df/1
  a_d/1 -> feedback filter/1(a_d)
  Unit Delay/1 -> feedback filter/3(a_df_1)

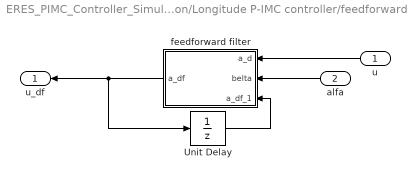
== system ERES_PIMC_Controller_Simulation/Longitude P-IMC controller/feedforward filter ==
  u : Inport
  alfa : Inport  Port=2
  Unit Delay : UnitDelay  SampleTime=-1
  feedforward filter : MATLAB Function  TreatAsAtomicUnit=on
  u_df : Outport
  wires:
  alfa/1 -> feedforward filter/2(belta)
  feedforward filter/1(a_df) -> Unit Delay/1, u_df/1
  u/1 -> feedforward filter/1(a_d)
  Unit Delay/1 -> feedforward filter/3(a_df_1)

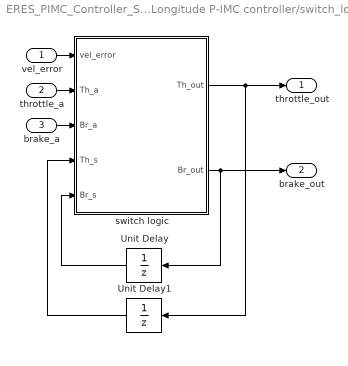
== system ERES_PIMC_Controller_Simulation/Longitude P-IMC controller/switch_logic ==
  vel_error : Inport
  throttle_a : Inport  Port=2
  brake_a : Inport  Port=3
  Unit Delay : UnitDelay  SampleTime=-1
  Unit Delay1 : UnitDelay  SampleTime=-1
  switch logic : MATLAB Function  TreatAsAtomicUnit=on
  throttle_out : Outport
  brake_out : Outport  Port=2
  wires:
  brake_a/1 -> switch logic/3(Br_a)
  switch logic/2(Br_out) -> brake_out/1, Unit Delay/1
  switch logic/1(Th_out) -> throttle_out/1, Unit Delay1/1
  Unit Delay1/1 -> switch logic/4(Th_s)
  Unit Delay/1 -> switch logic/5(Br_s)
  throttle_a/1 -> switch logic/2(Th_a)
  vel_error/1 -> switch logic/1(vel_error)

== system ERES_PIMC_Controller_Simulation/mass_estimateV1.0/feedforward filter ==
  u : Inport
  alfa : Inport  Port=2
  Unit Delay : UnitDelay  SampleTime=-1
  feedforward filter : MATLAB Function  TreatAsAtomicUnit=on
  u_df : Outport
  wires:
  alfa/1 -> feedforward filter/2(belta)
  feedforward filter/1(a_df) -> Unit Delay/1, u_df/1
  u/1 -> feedforward filter/1(a_d)
  Unit Delay/1 -> feedforward filter/3(a_df_1)

== system ERES_PIMC_Controller_Simulation/mass_estimateV1.0/feedforward filter1 ==
  u : Inport
  alfa : Inport  Port=2
  Unit Delay : UnitDelay  SampleTime=-1
  feedforward filter : MATLAB Function  TreatAsAtomicUnit=on
  u_df : Outport
  wires:
  Unit Delay/1 -> feedforward filter/3(a_df_1)
  u/1 -> feedforward filter/1(a_d)
  feedforward filter/1(a_df) -> u_df/1, Unit Delay/1
  alfa/1 -> feedforward filter/2(belta)

== system ERES_PIMC_Controller_Simulation/mass_estimateV2.0/M_Trans_filter1 ==
  M_in : Inport
  Scope3 : Scope  NumInputPorts=2
  feedforward filter1 : Subsystem
  slope_compen1 : Constant  Value=0.98
  M_Out : Outport
  wires:
  feedforward filter1/1(u_df) -> Scope3/1, M_Out/1
  slope_compen1/1 -> feedforward filter1/2(alfa)
  M_in/1 -> Scope3/2, feedforward filter1/1(u)

== system ERES_PIMC_Controller_Simulation/mass_estimateV2.0/feedforward filter ==
  u : Inport
  alfa : Inport  Port=2
  Unit Delay : UnitDelay  SampleTime=-1
  feedforward filter : MATLAB Function  TreatAsAtomicUnit=on
  u_df : Outport
  wires:
  Unit Delay/1 -> feedforward filter/3(a_df_1)
  u/1 -> feedforward filter/1(a_d)
  feedforward filter/1(a_df) -> u_df/1, Unit Delay/1
  alfa/1 -> feedforward filter/2(belta)

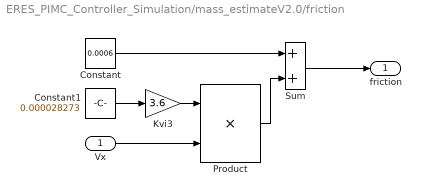
== system ERES_PIMC_Controller_Simulation/mass_estimateV2.0/friction ==
  Vx : Inport
  Constant : Constant  Value=0.0006
  Constant1 : Constant  Value=0.000028273
  Kvi3 : Gain  Gain=3.6
  Product : Product
  Sum : Sum
  friction : Outport
  wires:
  Vx/1 -> Product/2
  Sum/1 -> friction/1
  Constant1/1 -> Kvi3/1
  Product/1 -> Sum/2
  Constant/1 -> Sum/1
  Kvi3/1 -> Product/1

== system ERES_PIMC_Controller_Simulation/mass_estimateV3.0/M_Trans_filter1 ==
  M_in : Inport
  Scope3 : Scope  NumInputPorts=2
  feedforward filter1 : Subsystem
  slope_compen1 : Constant  Value=0.98
  M_Out : Outport
  wires:
  M_in/1 -> feedforward filter1/1(u), Scope3/2
  slope_compen1/1 -> feedforward filter1/2(alfa)
  feedforward filter1/1(u_df) -> M_Out/1, Scope3/1

== system ERES_PIMC_Controller_Simulation/mass_estimateV3.0/feedforward filter ==
  u : Inport
  alfa : Inport  Port=2
  Unit Delay : UnitDelay  SampleTime=-1
  feedforward filter : MATLAB Function  TreatAsAtomicUnit=on
  u_df : Outport
  wires:
  alfa/1 -> feedforward filter/2(belta)
  feedforward filter/1(a_df) -> Unit Delay/1, u_df/1
  u/1 -> feedforward filter/1(a_d)
  Unit Delay/1 -> feedforward filter/3(a_df_1)

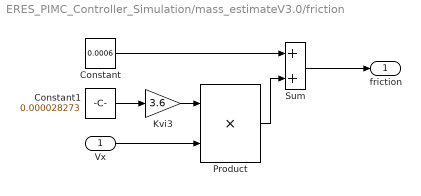
== system ERES_PIMC_Controller_Simulation/mass_estimateV3.0/friction ==
  Vx : Inport
  Constant : Constant  Value=0.0006
  Constant1 : Constant  Value=0.000028273
  Kvi3 : Gain  Gain=3.6
  Product : Product
  Sum : Sum
  friction : Outport
  wires:
  Kvi3/1 -> Product/1
  Constant/1 -> Sum/1
  Product/1 -> Sum/2
  Constant1/1 -> Kvi3/1
  Sum/1 -> friction/1
  Vx/1 -> Product/2

== system ERES_PIMC_Controller_Simulation/mass_estimateV2.0/M_Trans_filter1/feedforward filter1 ==
  u : Inport
  alfa : Inport  Port=2
  Unit Delay : UnitDelay  SampleTime=-1
  feedforward filter : MATLAB Function  TreatAsAtomicUnit=on
  u_df : Outport
  wires:
  Unit Delay/1 -> feedforward filter/3(a_df_1)
  u/1 -> feedforward filter/1(a_d)
  feedforward filter/1(a_df) -> u_df/1, Unit Delay/1
  alfa/1 -> feedforward filter/2(belta)

== system ERES_PIMC_Controller_Simulation/mass_estimateV3.0/M_Trans_filter1/feedforward filter1 ==
  u : Inport
  alfa : Inport  Port=2
  Unit Delay : UnitDelay  SampleTime=-1
  feedforward filter : MATLAB Function  TreatAsAtomicUnit=on
  u_df : Outport
  wires:
  alfa/1 -> feedforward filter/2(belta)
  feedforward filter/1(a_df) -> Unit Delay/1, u_df/1
  u/1 -> feedforward filter/1(a_d)
  Unit Delay/1 -> feedforward filter/3(a_df_1)

== matlab function ERES_PIMC_Controller_Simulation/trucksim_output ==
  data: lateral_error output; roll output; X output; Y output; Heading output; u input; Vx output; angular_vel output; Ac output; F_air output; Iw_Dr_L1 output; Iw_Dr_L2 output; Iw_Dr_L3 output; Iw_Dr_L4 output; Iw_Dr_L5 output; Engine_rpm output; M_Eng_In output; M_EngOut output; M_Tc output; M_Trans output; pitch output; gear output
function [lateral_error,roll,X,Y,Heading,Vx,angular_vel,Ac,F_air,Iw_Dr_L1...
    ,Iw_Dr_L2,Iw_Dr_L3,Iw_Dr_L4,Iw_Dr_L5,Engine_rpm,M_Eng_In,M_EngOut,M_Tc,M_Trans,pitch,gear]  = fcn(u)

%牵引车信息
X=u(1);
Y=u(2);
Yaw=u(3);
vx=u(4)/3.6;
vy=u(5)/3.6;
Avz=u(6);% unit:deg/s
Heading = Yaw/57.3;  
Vx = vx;%unit:m/s
angular_vel = Avz/57.3;%unit:rad/s
%半挂车信息
X2=u(7);
Y2=u(8);
Yaw2=u(9);
Avz2=u(10);

roll=u(11)/57.3;%unit rad
roll2=u(12);
hitch=u(13);
Ac = u(14) * 9.8;
lateral_error = u(15);
F_air = u(16);% kongqi zuli
Iw_Dr_L1 = u(17);%wheel inertia
Iw_Dr_L2 = u(18);
Iw_Dr_L3 = u(19);
Iw_Dr_L4 = u(20);
Iw_Dr_L5 = u(21);
Iw_Dr_L6 = u(22);
M_Eng_In = u(23);%engin torque
M_EngOut = u(24);
M_Tc = u(25);
M_Trans = u(26);
pitch = u(27) / 57.3;%unit rad
Engine_rpm = u(28) ;
gear = u(29);

% 车辆坐标系到大地坐标系的转换
% psi1=Yaw/57.3;
% dpsi1=Avz/57.3;
% 
% L=[cos(psi1) -sin(psi1);
%       sin(psi1) cos(psi1)];
% 
% dX=vx*cos(psi1)-vy*sin(psi1);
% dY=vx*sin(psi1)+vy*cos(psi1);%大地系下的速度

== matlab function ERES_PIMC_Controller_Simulation/mass_estimateV1.0/mass identification1 ==
  data: mass output; Fc input; theta input; Ft input; xi input; mass_k_1 input; p_k_1 input; K_k_1 input; P output; K output
function [mass,P,K] = fcn(Fc,theta,Ft,xi,mass_k_1,p_k_1,K_k_1)
% Fc = 0;theta = 0;Ft = 0;
na = 1;nb = 1;d = 3; %structure parameters
uk = 0;%initial value of system input
yk = 0;%initial value of system output
L = 1;
g = 9.8;%unit:m/s^2
w = 0.998;
%theta = 0;% slope of the road,unit:degree or rad?

% xi = sqrt(0.1) * randn(L,1);%white noise 
if theta >= 0 
    i = -sin(theta); 
else
    i = sin(theta); 
end
% i = -sin(theta); 
phi = g * i;

Fg = (Fc - Ft - xi) * -1;
% mass = 0;% initial value of the object to be estimated
% persistent mass_last;
% mass_last = 0;
% P = 10^6 * eye(na - 1 + nb - 1 + 1);
% Fg = phi * m + xi; % y(k) = phi(k)' * theta + xi 标准的最小二乘形式
% mass_data 

% RLS algorithm
K = p_k_1 * phi / (w + phi' * p_k_1 * phi);
% mass = mass_last + K * (Fg - phi' * mass_last);
mass = mass_k_1 + K * (Fg - phi' * mass_k_1);
P =1 / w * (eye(na - 1 + nb - 1 + 1) - K * phi') * p_k_1;

% mass_last = mass;

== matlab function ERES_PIMC_Controller_Simulation/Longitude P-IMC controller/feedback filter/feedback filter ==
  data: a_d input; belta input; a_df output; a_df_1 input
function a_df = fcn(a_d,belta,a_df_1)

a_df = belta * a_df_1 + ( 1 - belta) * a_d;

== matlab function ERES_PIMC_Controller_Simulation/mass_estimateV1.0/mass identification2 ==
  data: mass output; ac input; theta input; Ft input; noise input; w input; mass_k_1 input; p_k_1 input; K_k_1 input; P output; K output; gi output; phi output; err output; Fg output
function [mass,P,K,gi,phi,err,Fg] = fcn(ac,theta,Ft,noise,w,mass_k_1,p_k_1,K_k_1)
% Fc = 0;theta = 0;Ft = 0;
na = 1;nb = 1;d = 3; %structure parameters
uk = 0;%initial value of system input
yk = 0;%initial value of system output
L = 1;
g = 9.8;%unit:m/s^2
% w = 0.998;
%theta = 0;% slope of the road,unit:degree or rad?

% xi = sqrt(0.1) * randn(L,1);%white noise 
% if theta >= 0 
%     i = sin(theta); 
% else
%     i = -sin(theta); 
% end
i = sin(theta); 
gi = g*i;
if (ac<0.1) && (ac >0)
    ac = 0.05;
end
if  (ac<0.0) && (ac >-0.1)
         ac = -0.05;
end
phi = g * i +ac  ;%- noise
% phi = g * i  - noise;

% Fg = (Fc - Ft - noise) * -1;
% Fg = -1 * (ac * 20000 - Ft) ;
% Fg = -1 * ( Ft) ;
if ac >0 && Ft < 0
    Ft = -Ft;
elseif ac <0 && Ft >0
    Ft = -Ft;
else
    
end

Fg = 1 * ( Ft) + noise ;
% mass = 0;% initial value of the object to be estimated
% persistent mass_last;
% mass_last = 0;
% P = 10^6 * eye(na - 1 + nb - 1 + 1);
% Fg = phi * m + xi; % y(k) = phi(k-1)' * theta + xi 标准的最小二乘形式
% mass_k_1  = 10000; 

% RLS algorithm
err = Fg - phi' * mass_k_1;
% P =1 / w * (eye(na - 1 + nb - 1 + 1) - K * phi') * p_k_1;% covariance matrix
% K = p_k_1 * phi / (w + phi' * p_k_1 * phi);   %gain matrix
K = p_k_1 * phi / (w + phi' * p_k_1 * phi);   %gain matrix
% mass = mass_last + K * (Fg - phi' * mass_last);
mass = mass_k_1 + K * (Fg - phi' * mass_k_1);% Fg - phi' * mass_k_1 identification error
% P =1 / w * (eye(na - 1 + nb - 1 + 1) - K_k_1 * phi') * p_k_1;% covariance matrix
% P =1 / w * (eye(na - 1 + nb - 1 + 1) - K_k_1 * phi') * p_k_1;% covariance matrix
% P =1 / w * (p_k_1 - ( p_k_1 * phi * phi' *p_k_1) / ( w + phi' *  p_k_1 * phi)) ;
P =1 / w * (p_k_1 -  p_k_1 * phi  / ( w + phi' *  p_k_1 * phi) * phi' *p_k_1) ;

% if mass <=0
%     mass = 0;
% end

% mass_last = mass;

== matlab function ERES_PIMC_Controller_Simulation/Longitude P-IMC controller/feedforward filter/feedforward filter ==
  data: a_d input; belta input; a_df output; a_df_1 input
function a_df = fcn(a_d,belta,a_df_1)

a_df = belta * a_df_1 + ( 1 - belta) * a_d;

== matlab function ERES_PIMC_Controller_Simulation/Longitude P-IMC controller/alfa interpolate ==
  data: vel_error input; alfa output
function alfa = fcn(vel_error)

alfa_table = [0.01,0.108,0.206,0.304,0.402,0.5,0.598,0.696,0.794,0.892,0.99];
% belta_table = [0.01,0.108,0.206,0.304,0.402,0.5,0.598,0.696,0.794,0.892,0.99];
% vel_table = [25,22.51,20.02,17.53,15.04,12.55,10.06,7.57,5.08,2.59,0.1];
vel_table = [10.0000    8.0100    7.0200    6.5300    6.0400    5.0500    4.0600    3.0700    2.0800    1.0900    0.1000];

 alfa = interp1(vel_table,alfa_table,vel_error,'spline');
  if alfa< 0.01
     alfa = 0.01;
 elseif alfa >= 0.99
     alfa = 0.99;
 end

== matlab function ERES_PIMC_Controller_Simulation/eres_controller ==
  data: X input; Y input; heading input; vx input; K_expect output; fl_x input; fl_y input; fr_x input; fr_y input; num input; x0 input; y0 input; w1 input; w2 input; t_delay input; a_lateral_max input; steer_angle_limited input; K_expect_1 input; start_index output; start_index_1 input
function [K_expect,start_index]  = fcn(X,Y,heading,vx,fl_x,fl_y,fr_x,fr_y,num,x0,y0,w1,w2,t_delay,a_lateral_max,steer_angle_limited,K_expect_1,start_index_1)
%using arc for sampling
% q = floor((klmin - krmax) / delta_k);
p = num;
s = ones(30,1);
s_thresh = 1.2;
klmin = 0.000001;
krmax = 0.000001;
% num = 30;
% fprintf("x_max = %f",x_max);
x_max = 0.00000;
% fprintf("x_max = %f",x_max);
kmax = 1.5;
% klmin = -kmax;
% krmax = kmax;
max_deceleration = 6.0;

C_proximity = ones(num,1);
C_smooth = ones(num,1);
xp_ =  ones(num,1);
sp_ =  ones(num,1);
yp_ =  ones(num,1);
K_expect = 0.0; 
C_p = 0.000001;
C_cost = ones(num,1);
tmp = 0;
index = 1;
%% find the start index 
start_index = 1;
% fprintf("start_index_1 = %f\n",start_index_1);
% start_index = floor(X);

for i = 1:1:length(fl_x)
    if(X < fl_x( i )) || (X< fr_x( i ))
        start_index = i - 1;
        break;
    end
%     break;
end

if start_index <= 1
    start_index = 1;
end

%% convert the coordinates to vehicle coordinate system
fl_x_tmp = zeros(30,1);
fl_y_tmp = zeros(30,1);
fr_x_tmp = zeros(30,1);
fr_y_tmp = zeros(30,1);
for i=1:num
%     fl_xe(i) =fl_x( start_index+i-1 ) ;
    fl_x_tmp(i) = fl_x(start_index + i -1 );
    fl_y_tmp(i) = fl_y(start_index + i -1 );
    fr_x_tmp(i) = fr_x(start_index + i -1 );
    fr_y_tmp(i) = fr_y(start_index + i -1 );
    
end

% left and right line coordinates in global coodinate system
% fl_x_tmp = fl_x( start_index:start_index + num );
% fl_y_tmp = fl_y( start_index:start_index + num );
% fr_x_tmp = fr_x( start_index:start_index + num );
% fr_y_tmp = fr_y( start_index:start_index + num );
% left and right line coordinates in vehicle coodinate system
if X <0
    X = 0;
end
fl_xe = (fl_x_tmp - X) * cos (heading) + (fl_y_tmp - Y) * sin(heading);
fl_ye = (fl_y_tmp - Y) * cos (heading) - (fl_x_tmp - X) * sin(heading);

fr_xe = (fr_x_tmp - X) * cos (heading) + (fr_y_tmp - Y) * sin(heading);
fr_ye = (fr_y_tmp - Y) * cos (heading) - (fr_x_tmp - X) * sin(heading);


%% search control space
% fresh kmax and s_thresh every cycle
% fprintf("vx = %f \n",vx);
% fprintf("a_lateral_max / vx^2 = %f \n",a_lateral_max / vx^2);
% kmax = min((tan(steer_angle_limited/57.3))/4.75 , a_lateral_max / vx^2);
% kmax = min((tan(steer_angle_limited)/57.3)/4.75 , 1.5);
kmax = (tan(steer_angle_limited/57.3))/4.75 ;
% kmax = 1.5;
klmin = kmax;
krmax = -kmax;

% s_thresh = vx ^2 / (2 * max_deceleration) + vx * t_delay;
s_thresh =10;

% fprintf("kmax = %f \n",kmax);
% fprintf("s_thresh = %f \n",s_thresh);

kl = 2 .*  fl_ye ./ (fl_ye.^2 + fl_xe.^2);
kr = 2 .* fr_ye ./ (fr_ye.^2 + fr_xe.^2);

%  the arc length
sl  = 2 .* asin(fl_ye ./ sqrt(fl_xe.^2 + fl_ye.^2)) ./ kl;
sr = 2 .* asin(fr_ye ./ sqrt(fr_xe.^2 + fr_ye.^2)) ./ kr;

for i=1:num 
    s(i)=max(sl(i),sr(i));
%     fprintf("kl (%f) = %f \n",i,kl(i));
%     fprintf("kr (%f) = %f \n",i,kr(i));
%     
%     fprintf("fr_x (%f) = %f \n",i,fr_x(i));
%     fprintf("fr_y (%f) = %f \n",i,fr_y(i));
%     
    
%     if (s(i)<s_thresh)
%         continue;
%     else
%         if (kl(i)<klmin)
%             klmin=kl(i);
% %             fprintf("kl (%f) = %f \n",i,kl(i));
%         end
%         
%         if (kr(i)>-kmax)
%             krmax=kr(i);
%         end
%         
%         x_max=fl_xe(i);%x_max
% %         fprintf("x_max = %f \n",x_max);
%         kr(i)=krmax;
%         kl(i)=klmin;
% %         fprintf("kr (%f) = %f \n",i,kr(i));
%        
%     end
%     %
%     if (kl(i)<kr(i))
%             x_max=fl_xe(i-1);
%         break;
%     else
%         
%     end
%     x_max = 30;



    if kl(i) < kr(i)
        x_max = (i - 1);
        break;
    elseif s(i) < s_thresh
        continue;
    else
        if kl(i) < klmin
            klmin = kl( i );
        end
        
        if kr( i ) > krmax
            krmax = kr( i );
        end
        
        kr( i ) = krmax;
        kl( i ) = klmin;
        x_max = i;
    end
 





end
fprintf("x_max = %f \n",x_max);
%% choose best arc
fprintf("kr(x_max) = %f \n",kr(x_max));
fprintf("kl(x_max) = %f \n",kl(x_max));
% kp = linspace(krmax,klmin,p);
kp = linspace(kr(x_max),kl(x_max),p);
for j = 1:1:(p )
%     fprintf("kp (%f) = %f \n",j,kp(j));
    
    xp_ = linspace(0,x_max,p);
    sp_ = asin(kp(j)*(xp_-x0))/kp(j);
    yp_ = -1/kp(j)*cos(kp(j)*sp_)+1/kp(j)+y0;

    for n = 1:1:length(num)
        tmp = min(abs(yp_( n ) - fl_ye(n)),abs(yp_(n ) - fr_ye(n)));
        C_p = C_p + tmp;
%         fprintf('C_p = %f \n',C_p);
    end

    C_proximity(j) = 1 / C_p;
    C_smooth(j) = (kp(j) - K_expect_1)^2;
    C_p = 0.000001;           
%             plot(xp_,yp_,'y*');%

end

C_cost = w1* C_proximity + w2 * C_smooth;
C_cost_min = C_cost(1);
for m = 1:1:length(C_cost)
    if C_cost(m) <= C_cost_min
        C_cost_min = C_cost(m);
        K_expect = kp(m);
        index = m;
    end 
end

% fprintf('K_expect = %f \n',K_expect);
% fprintf('index = %f \n',index);  


 xy=linspace(0,x_max,100);
 sy=asin(K_expect_1*(xy-x0))/K_expect_1;
 fy=-1/K_expect_1*cos(K_expect_1*sy)+1/K_expect_1+y0;
 plot(xy,fy,'r*')

== matlab function ERES_PIMC_Controller_Simulation/Longitude P-IMC controller/belta interpolate ==
  data: vel_error input; belta output
function belta= fcn(vel_error)

% belta_table = [0.01,0.108,0.206,0.304,0.402,0.5,0.598,0.696,0.794,0.892,0.99];
belta_table = [0.05,0.308,0.356,0.394,0.402,0.5,0.598,0.696,0.794,0.892,0.19];

% vel_table = [25,22.51,20.02,17.53,15.04,12.55,10.06,7.57,5.08,2.59,0.1];
% vel_table = [10.0000    9.0100    8.0200    7.0300    6.0400    5.0500    4.0600    3.0700    2.0800    1.0900    0.1000];
% vel_table = [10.0000    7.0100    6.0200    5.0300    4.5400    4.0500    3.5600    3.0700    2.0800    1.0900    0.001000];
vel_table = [10.0000    7.0100    6.0200    5.0300    4.5400    4.0500    3.5600    3.0700    2.0800    1.0900    0.1000];
% vel_table = [0.1000    1.0900    2.0800     3.0700   3.5600    4.0500    4.5400     5.0300      6.0200    7.0100   10.0000];

 belta = interp1(vel_table,belta_table,vel_error,'spline');
 if belta< 0.01
     belta = 0.01;
 elseif belta >= 0.99
     belta = 0.99;
 end

== matlab function ERES_PIMC_Controller_Simulation/steer_angle_2/steer_roll_compensation ==
  data: roll input; steer_roll_ output
function steer_roll_ = fcn(roll)

steer_roll_ = 9.8 * sin(roll) * 20.34 * 57.3;

== matlab function ERES_PIMC_Controller_Simulation/steer_angle_1/steer_compensation ==
  data: lateral_error input; steer_compensation output
function steer_compensation = fcn(lateral_error)

steer_compensation = 1 * lateral_error * 20.34 * 57.3;

== matlab function ERES_PIMC_Controller_Simulation/steer_angle ==
  data: steer_angle output; curvature input; steer_ratio input; wheel_base input
function steer_angle  = fcn(curvature,steer_ratio,wheel_base)
steer_angle = steer_ratio * atan(wheel_base * curvature) * 180 / pi;

== matlab function ERES_PIMC_Controller_Simulation/choose_vr ==
  data: Vr_points input; vr output; index output; index_1 input
function [vr,index] = fcn(Vr_points,index_1)
index = index_1 + 1;
vr = Vr_points(index + 1);
% fprintf("vr index = %f",index);

== matlab function ERES_PIMC_Controller_Simulation/Longitude P-IMC controller/switch_logic/switch logic ==
  data: vel_error input; Th_out output; Th_a input; Br_a input; Th_s input; Br_s input; Br_out output
function [Th_out,Br_out] = fcn(vel_error,Th_a,Br_a,Th_s,Br_s)
threshold = 0.01;
Ev = 0.1;
if vel_error < -Ev % deceleration
    if(Th_s > threshold)% throttle control
        Th_out = Th_a;
        Br_out = 0;
    else% brake control
        Th_out = 0;
        Br_out = Br_a;
    end
    
else
    if vel_error > Ev % acceleration
        if(Br_s > threshold) % brake control
            Th_out = 0;
            Br_out = Br_a;
        else % throttle control
            Th_out = Th_a;
            Br_out = 0;
        end
    else % keep region
        if Br_s > threshold
            Th_out = 0;
            Br_out = Br_a;
        else
            if Th_s > threshold
                Th_out = Th_a;
                Br_out = 0; 
            else
                Th_out = 0;
                Br_out = 0;
            end
        end
    end
end

== matlab function ERES_PIMC_Controller_Simulation/mass_estimateV1.0/feedforward filter/feedforward filter ==
  data: a_d input; belta input; a_df output; a_df_1 input
function a_df = fcn(a_d,belta,a_df_1)

a_df = belta * a_df_1 + ( 1 - belta) * a_d;
